simulink model "sistema_inic_maberta"  (Simulink 5.0)
settings: Solver=ode45  StartTime=0.0  StopTime=60  RelTol=1e-3
libraries: simulink x2
settings Model: LastModifiedBy=Lu

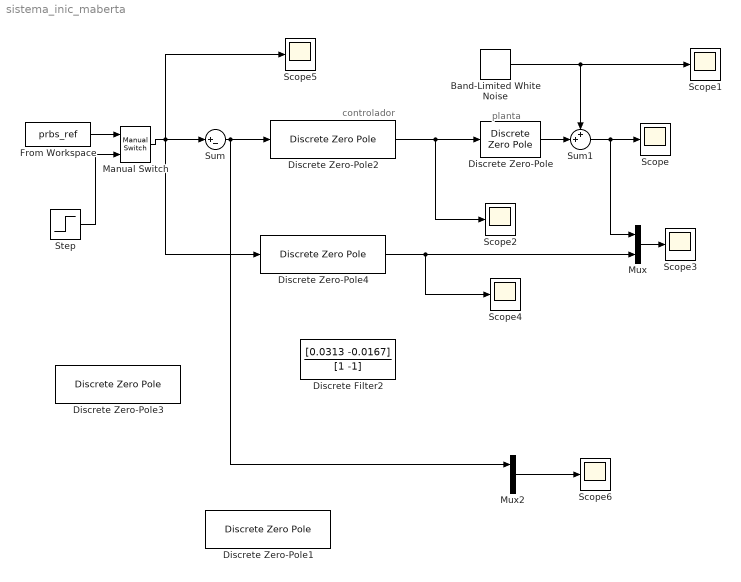
== system sistema_inic_maberta ==
  note: planta
  note: controlador
  Band-Limited White Noise : simulink/Sources/Band-Limited White Noise  Cov=[0.01]  Ts=1  seed=[23341]
  Discrete Zero-Pole : DiscreteZeroPole  Zeros=[]  Poles=[0.2 0.3]  Gain=10
  Discrete Zero-Pole1 : DiscreteZeroPole  Zeros=[0.2 0.4]  Poles=[0.9 -0.4]  Gain=0.035
  Discrete Zero-Pole2 : DiscreteZeroPole  Zeros=[0.3 0.2]  Poles=[1 -0.2]  Gain=0.035
  Discrete Zero-Pole3 : DiscreteZeroPole  Zeros=[0.3 0.2]  Poles=[1 -0.2]  Gain=0.035
  Discrete Zero-Pole4 : DiscreteZeroPole  Zeros=[]  Poles=[0.5 0.3]  Gain=0.35
  Discrete Filter2 : DiscreteFilter  Numerator=[0.0313 -0.0167]  Denominator=[1 -1]
  From Workspace : FromWorkspace  VariableName=prbs_ref  SampleTime=0
  Manual Switch : simulink/Signal Routing/Manual Switch  sw=1  action=0
  Mux : Mux  Inputs=2
  Mux2 : Mux  Inputs=2
  Scope{,1..6} (7 alike) : Scope
      Scope settings: SaveName=y_scope  DataFormat=Array
      Scope1 settings: SaveName=y_scope2  DataFormat=Array
      Scope2 settings: SaveName=u_scope  DataFormat=Array
      Scope3 settings: SaveName=y_scope1  DataFormat=Array
      Scope4 settings: SaveName=y_scope_mod  DataFormat=Array
      Scope5 settings: SaveName=ref_scope  DataFormat=Array  SampleInput=on  SampleTime=1
      Scope6 settings: SaveName=y_scope3  DataFormat=Array  SampleTime=1
  Step : Step  Time=0  SampleTime=0
  Sum : Sum  Inputs=|+-  SaturateOnIntegerOverflow=on
  Sum1 : Sum  Inputs=++|  SaturateOnIntegerOverflow=on
  wires:
  Mux/1 -> Scope3/1
  Discrete Zero-Pole4/1 -> Mux/2, Scope4/1
  Mux2/1 -> Scope6/1
  Sum/1 -> Mux2/1, Discrete Zero-Pole2/1
  ? -> Mux2/2
  Discrete Zero-Pole/1 -> Sum1/2
  Sum1/1 -> Scope/1, Mux/1
  Band-Limited White Noise/1 -> Scope1/1, Sum1/1
  Manual Switch/1 -> Sum/1, Scope5/1, Discrete Zero-Pole4/1
  Step/1 -> Manual Switch/2
  From Workspace/1 -> Manual Switch/1
  Discrete Zero-Pole2/1 -> Discrete Zero-Pole/1, Scope2/1
